simulink model "advanced_normal_buck_converter"  (R2023b)
settings: Solver=VariableStepAuto  StartTime=0.0  StopTime=0.2  FixedStep=0.0002  MaxStep=0.0001  RelTol=1e-3
undefined symbols (not defined in the file or in its folder): Acid, Lead
libraries: spsDiodeLib x8, spsSeriesRLCBranchLib x7, spsCurrentMeasurementLib x4, spsVoltageMeasurementLib x4, spsACVoltageSourceLib x3, spsBatteryLib x1, spsGroundLib x1, spsMosfetLib x1, spsPWMGeneratorDCDCLib x1, sps_lib x1
settings Model: Creator=Msi  LastModifiedBy=Msi

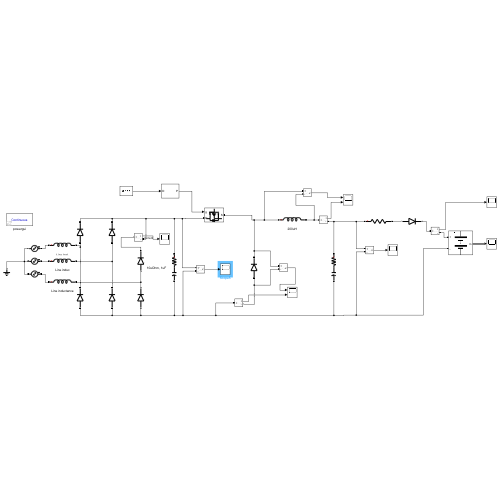
[thumbnail: Simulink's stored preview of the top-level diagram]
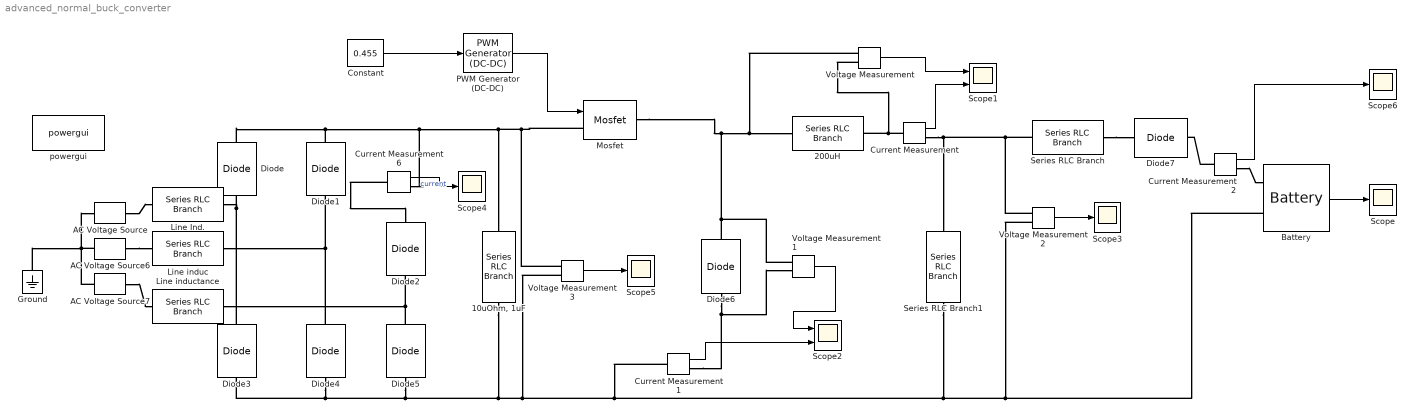
== system advanced_normal_buck_converter ==
  "10uOhm, 1uF" : spsSeriesRLCBranchLib/Series RLC Branch  LConnTagsString=__new0  RConnTagsString=__new0  BranchType=RC  Resistance=1e-5  Inductance=1e-3  SetiL0=off  InitialCurrent=0  Capacitance=10e-6  Setx0=off  InitialVoltage=0  Measurements=None
  200uH : spsSeriesRLCBranchLib/Series RLC Branch  LConnTagsString=__new0  RConnTagsString=__new0  BranchType=L  Resistance=1  Inductance=470e-6  SetiL0=off  InitialCurrent=0  Capacitance=1e-6  Setx0=off  InitialVoltage=0  Measurements=None
  AC Voltage Source : spsACVoltageSourceLib/AC Voltage Source  Amplitude=25*sqrt(2)/sqrt(3)  Phase=0  Frequency=50  SampleTime=0  Measurements=None  BusType=swing  Pref=10e3  Qref=0  Qmin=-inf  Qmax=+inf
  AC Voltage Source6 : spsACVoltageSourceLib/AC Voltage Source  Amplitude=25*sqrt(2)/sqrt(3)  Phase=120  Frequency=50  SampleTime=0  Measurements=None  BusType=swing  Pref=10e3  Qref=0  Qmin=-inf  Qmax=+inf
  AC Voltage Source7 : spsACVoltageSourceLib/AC Voltage Source  Amplitude=25*sqrt(2)/sqrt(3)  Phase=240  Frequency=50  SampleTime=0  Measurements=None  BusType=swing  Pref=10e3  Qref=0  Qmin=-inf  Qmax=+inf
  Battery : spsBatteryLib/Battery  BatType=Lead-Acid  ShowTempParam=off  ThermalPreset=no  ShowAgeParam=off  NomV=12  NomQ=100  SOC=40  Batt_Tr=30  PresetModel=on  MaxQ=104.1667  MinV=9  FullV=13.0658  Dis_rate=20  R=0.0012  Normal_OP=31.0278  expZone="[12.2171     0.333333]"  current=[6.5 13 32.5]  Units=Time  Tci=20  NomT=20  T2=-30  MaxQ2=4.8  FullV2=7.1  Normal_OP2=5.655  expZone2="[6.58           1]"  Rca=0.6  ti=2000  Dp=0  Neq0=0  Tsim=1e6  Ta1=25  Qeol=5.4*0.9  Reol=0.013333*1.2  Char_age=[2.3478, 3]  Dis_age=[2.3478, 10]  N1=1500  N2=10500  N3=1000  N4=1400  Ta2=45  N5=950
  Constant : Constant  Value=0.455
  Current Measurement{,1..2,6} (4 alike) : spsCurrentMeasurementLib/Current Measurement  PhasorSimulation=off  OutputType=Complex  PSBequivalent=0
  Diode{,1..7} (8 alike) : spsDiodeLib/Diode  Ron=0.001  Lon=0  Vf=0.8  IC=0  UseSnubber=0  Rs=0  Cs=0  Measurements=off
  Ground : spsGroundLib/Ground  LConnTagsString=a
  Line Ind. : spsSeriesRLCBranchLib/Series RLC Branch  LConnTagsString=__new0  RConnTagsString=__new0  BranchType=L  Resistance=1  Inductance=200e-6  SetiL0=off  InitialCurrent=0  Capacitance=1e-6  Setx0=off  InitialVoltage=0  Measurements=None
  Line induc : spsSeriesRLCBranchLib/Series RLC Branch  LConnTagsString=__new0  RConnTagsString=__new0  BranchType=L  Resistance=1  Inductance=200e-6  SetiL0=off  InitialCurrent=0  Capacitance=1e-6  Setx0=off  InitialVoltage=0  Measurements=None
  Line inductance : spsSeriesRLCBranchLib/Series RLC Branch  LConnTagsString=__new0  RConnTagsString=__new0  BranchType=L  Resistance=1  Inductance=200e-6  SetiL0=off  InitialCurrent=0  Capacitance=1e-6  Setx0=off  InitialVoltage=0  Measurements=None
  Mosfet : spsMosfetLib/Mosfet  Ron=0.1  Lon=0  Rd=0.01  Vfd=0  IC=0  Rs=1e5  Cs=inf  Measurements=off
  PWM Generator (DC-DC) : spsPWMGeneratorDCDCLib/PWM Generator (DC-DC)  Fsw=50000  Ts=0
  Scope{,3..6} (5 alike) : Scope
  Scope1 : Scope  NumInputPorts=2
  Scope2 : Scope  NumInputPorts=2
  Series RLC Branch : spsSeriesRLCBranchLib/Series RLC Branch  LConnTagsString=__new0  RConnTagsString=__new0  BranchType=R  Resistance=0.1  Inductance=1e-3  SetiL0=off  InitialCurrent=0  Capacitance=1e-6  Setx0=off  InitialVoltage=0  Measurements=None
  Series RLC Branch1 : spsSeriesRLCBranchLib/Series RLC Branch  LConnTagsString=__new0  RConnTagsString=__new0  BranchType=RC  Resistance=0.25  Inductance=1e-3  SetiL0=off  InitialCurrent=0  Capacitance=10e-6  Setx0=off  InitialVoltage=0  Measurements=None
  Voltage Measurement{,1..3} (4 alike) : spsVoltageMeasurementLib/Voltage Measurement  PhasorSimulation=off  OutputType=Complex  PSBequivalent=0
  powergui : sps_lib/powergui  Priority=1  SimulationMode=Continuous  SampleTime=0.0002  frequency=60  Iterations=50  frequencyindice=50  Pbase=100e6  ErrMax=1e-4  UnitsV=kV  UnitsW=MW  buscounter=0  FunctionMessages=off  echomessages=off  EnableUseOfTLC=off  CurrentSourceSwitches=off  DisableSnubberDevices=off  DisableRonSwitches=off  DisableVfSwitches=off  DisplayEquations=off  AutomaticDiscreteSolvers=off  SolverType=Tustin/Backward Euler (TBE)  Interpol=off  ExternalGateDelay=off  methode=off  Ts=100  x0status=blocks  SPID=on  SwTol=0  HookPort=off  NonlinearTolerance=1e-4  nMaxIteration=100  ContinueOnMaxIteration=off  RestoreLinks=warning  ResistiveCurrentMeasurement=off  Frange=[0:2:500]  Ylog=off  Xlog=on  ShowGrid=off  save=off  variable=ZData  structure=0  ZoomFFT=off  StartTime=0.0  cycles=1  DisplayStyle=1  fundamental=60  FreqAxis=off  MaxFrequency=1000  frequencyindicesteady=1  RmsSteady=1  display=off
  wires:
  Battery/1 -> Scope/1
  Constant/1 -> PWM Generator (DC-DC)/1
  PWM Generator (DC-DC)/1 -> Mosfet/1
  Voltage Measurement/1 -> Scope1/1
  Current Measurement/1 -> Scope1/2
  Voltage Measurement1/1 -> Scope2/1
  Current Measurement1/1 -> Scope2/2
  Voltage Measurement2/1 -> Scope3/1
  Current Measurement6/1 -> Scope4/1  "current"
  Voltage Measurement3/1 -> Scope5/1
  Current Measurement2/1 -> Scope6/1
  connections:
  AC Voltage Source7/LConn1 -- Ground/LConn1 -- AC Voltage Source6/LConn1 -- AC Voltage Source/LConn1
  Diode3/RConn1 -- Line Ind./RConn1 -- Diode/LConn1
  Diode4/RConn1 -- Line induc/RConn1 -- Diode1/LConn1
  Diode/RConn1 -- Diode1/RConn1 -- Current Measurement6/RConn1 -- Voltage Measurement3/LConn1 -- Mosfet/LConn1 -- "10uOhm, 1uF"/LConn1
  Diode3/LConn1 -- Voltage Measurement3/LConn2 -- Voltage Measurement2/LConn2 -- Battery/LConn2 -- Series RLC Branch1/RConn1 -- Current Measurement1/LConn1 -- "10uOhm, 1uF"/RConn1 -- Diode5/LConn1 -- Diode4/LConn1
  Diode5/RConn1 -- Line inductance/RConn1 -- Diode2/LConn1
  Current Measurement6/LConn1 -- Diode2/RConn1
  Mosfet/RConn1 -- Voltage Measurement1/LConn1 -- Diode6/RConn1 -- Voltage Measurement/LConn1 -- 200uH/LConn1
  Voltage Measurement2/LConn1 -- Current Measurement/RConn1 -- Series RLC Branch1/LConn1 -- Series RLC Branch/LConn1
  Voltage Measurement/LConn2 -- Current Measurement/LConn1 -- 200uH/RConn1
  Diode6/LConn1 -- Voltage Measurement1/LConn2 -- Current Measurement1/RConn1
  AC Voltage Source7/RConn1 -- Line inductance/LConn1
  AC Voltage Source6/RConn1 -- Line induc/LConn1
  AC Voltage Source/RConn1 -- Line Ind./LConn1
  Series RLC Branch/RConn1 -- Diode7/LConn1
  Current Measurement2/LConn1 -- Diode7/RConn1
  Current Measurement2/RConn1 -- Battery/LConn1
